simulink library "Arithmetic_Operations_Lib"  (Simulink 8.7)
settings: Solver=ode45  StartTime=0.0  StopTime=10.0  RelTol=1e-3
libraries: Arithmetic_Operations_Lib x56, commutil2 x8
settings Model: Creator=uzivatel  LastModifiedBy=Jozko Mrkvicka

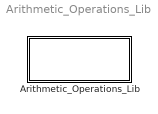
== system Arithmetic_Operations_Lib ==
  Arithmetic_Operations_Lib : Subsystem

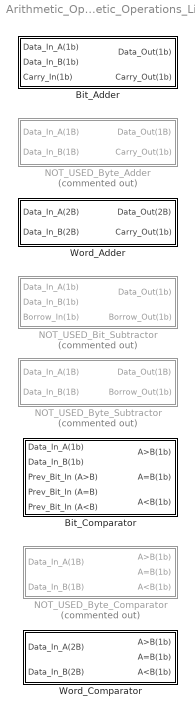
== system Arithmetic_Operations_Lib/Arithmetic_Operations_Lib ==
  Bit_Adder : Subsystem
  Bit_Comparator : Subsystem
  NOT_USED_Bit_Subtractor : Subsystem  Commented=on
  NOT_USED_Byte_Adder : Subsystem  Commented=on
  NOT_USED_Byte_Comparator : Subsystem  Commented=on
  NOT_USED_Byte_Subtractor : Subsystem  Commented=on
  Word_Adder : Subsystem
  Word_Comparator : Subsystem

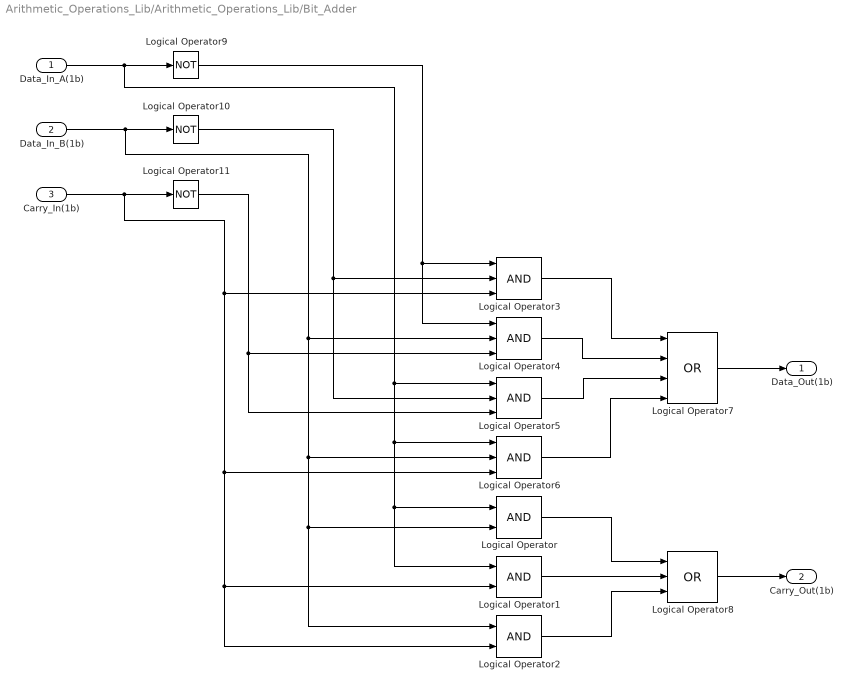
== system Arithmetic_Operations_Lib/Arithmetic_Operations_Lib/Bit_Adder ==
  Data_In_A(1b) : Inport
  Data_In_B(1b) : Inport  Port=2
  Carry_In(1b) : Inport  Port=3
  Logical Operator : Logic  IconShape=distinctive  AllPortsSameDT=off  OutDataTypeStr=boolean
  Logical Operator1 : Logic  IconShape=distinctive  AllPortsSameDT=off  OutDataTypeStr=boolean
  Logical Operator10 : Logic  Operator=NOT  Inputs=4  IconShape=distinctive  AllPortsSameDT=off  OutDataTypeStr=boolean
  Logical Operator11 : Logic  Operator=NOT  Inputs=4  IconShape=distinctive  AllPortsSameDT=off  OutDataTypeStr=boolean
  Logical Operator2 : Logic  IconShape=distinctive  AllPortsSameDT=off  OutDataTypeStr=boolean
  Logical Operator{3..6} (4 alike) : Logic  Inputs=3  IconShape=distinctive  AllPortsSameDT=off  OutDataTypeStr=boolean
  Logical Operator7 : Logic  Operator=OR  Inputs=4  IconShape=distinctive  AllPortsSameDT=off  OutDataTypeStr=boolean
  Logical Operator8 : Logic  Operator=OR  Inputs=3  IconShape=distinctive  AllPortsSameDT=off  OutDataTypeStr=boolean
  Logical Operator9 : Logic  Operator=NOT  Inputs=4  IconShape=distinctive  AllPortsSameDT=off  OutDataTypeStr=boolean
  Data_Out(1b) : Outport
  Carry_Out(1b) : Outport  Port=2
  wires:
  Logical Operator11/1 -> Logical Operator4/3, Logical Operator5/3
  Logical Operator10/1 -> Logical Operator3/2, Logical Operator5/2
  Logical Operator9/1 -> Logical Operator3/1, Logical Operator4/1
  Data_In_A(1b)/1 -> Logical Operator9/1, Logical Operator5/1, Logical Operator6/1, Logical Operator/1, Logical Operator1/1
  Data_In_B(1b)/1 -> Logical Operator10/1, Logical Operator4/2, Logical Operator6/2, Logical Operator/2, Logical Operator2/1
  Carry_In(1b)/1 -> Logical Operator11/1, Logical Operator3/3, Logical Operator6/3, Logical Operator1/2, Logical Operator2/2
  Logical Operator2/1 -> Logical Operator8/3
  Logical Operator1/1 -> Logical Operator8/2
  Logical Operator/1 -> Logical Operator8/1
  Logical Operator8/1 -> Carry_Out(1b)/1
  Logical Operator7/1 -> Data_Out(1b)/1
  Logical Operator6/1 -> Logical Operator7/4
  Logical Operator5/1 -> Logical Operator7/3
  Logical Operator4/1 -> Logical Operator7/2
  Logical Operator3/1 -> Logical Operator7/1

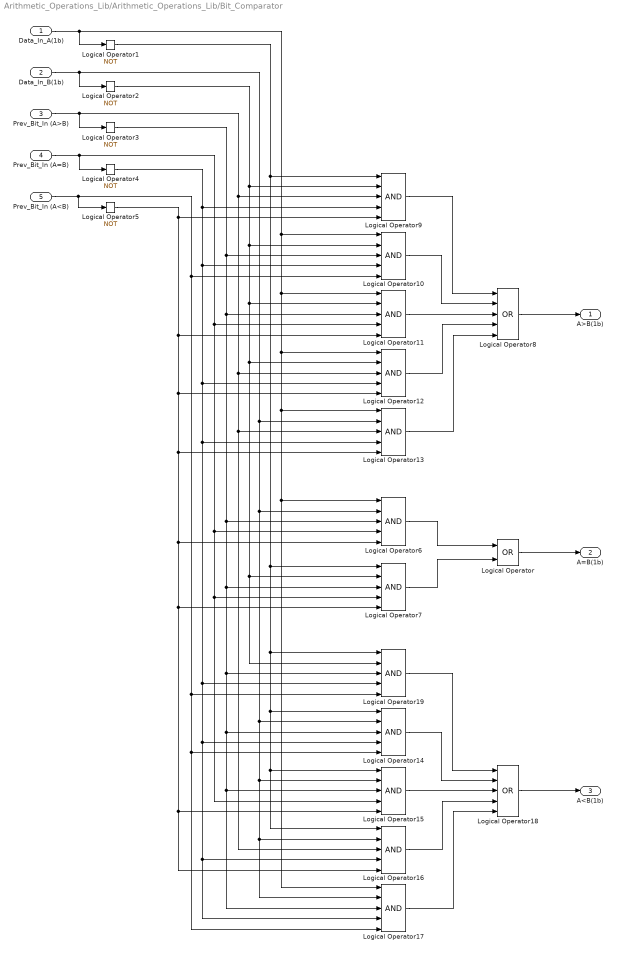
== system Arithmetic_Operations_Lib/Arithmetic_Operations_Lib/Bit_Comparator ==
  Data_In_A(1b) : Inport
  Data_In_B(1b) : Inport  Port=2
  Prev_Bit_In (A>B) : Inport  Port=3
  Prev_Bit_In (A=B) : Inport  Port=4
  Prev_Bit_In (A<B) : Inport  Port=5
  Logical Operator : Logic  Operator=OR  IconShape=distinctive  AllPortsSameDT=off  OutDataTypeStr=boolean
  Logical Operator{1..5} (5 alike) : Logic  Operator=NOT  IconShape=distinctive  AllPortsSameDT=off  OutDataTypeStr=boolean
  Logical Operator{6..7,9..17,19} (12 alike) : Logic  Inputs=5  IconShape=distinctive  AllPortsSameDT=off  OutDataTypeStr=boolean
  Logical Operator18 : Logic  Operator=OR  Inputs=5  IconShape=distinctive  AllPortsSameDT=off  OutDataTypeStr=boolean
  Logical Operator8 : Logic  Operator=OR  Inputs=5  IconShape=distinctive  AllPortsSameDT=off  OutDataTypeStr=boolean
  A>B(1b) : Outport
  A=B(1b) : Outport  Port=2
  A<B(1b) : Outport  Port=3
  wires:
  Logical Operator16/1 -> Logical Operator18/4
  Logical Operator17/1 -> Logical Operator18/5
  Logical Operator19/1 -> Logical Operator18/1
  Logical Operator15/1 -> Logical Operator18/3
  Logical Operator14/1 -> Logical Operator18/2
  Logical Operator4/1 -> Logical Operator9/4, Logical Operator10/4, Logical Operator12/4, Logical Operator13/4, Logical Operator19/4, Logical Operator14/4, Logical Operator17/4, Logical Operator16/4
  Data_In_A(1b)/1 -> Logical Operator10/1, Logical Operator11/1, Logical Operator12/1, Logical Operator13/1, Logical Operator6/1, Logical Operator17/1, Logical Operator1/1
  Logical Operator5/1 -> Logical Operator9/5, Logical Operator11/5, Logical Operator12/5, Logical Operator13/5, Logical Operator6/5, Logical Operator7/5, Logical Operator15/5, Logical Operator16/5
  Logical Operator18/1 -> A<B(1b)/1
  Logical Operator2/1 -> Logical Operator9/2, Logical Operator10/2, Logical Operator11/2, Logical Operator12/2, Logical Operator7/2, Logical Operator19/2
  Logical Operator1/1 -> Logical Operator9/1, Logical Operator7/1, Logical Operator19/1, Logical Operator14/1, Logical Operator15/1, Logical Operator16/1
  Logical Operator3/1 -> Logical Operator10/3, Logical Operator11/3, Logical Operator6/3, Logical Operator7/3, Logical Operator19/3, Logical Operator14/3, Logical Operator15/3, Logical Operator17/3
  Prev_Bit_In (A<B)/1 -> Logical Operator5/1, Logical Operator10/5, Logical Operator19/5, Logical Operator14/5, Logical Operator17/5
  Prev_Bit_In (A>B)/1 -> Logical Operator3/1, Logical Operator9/3, Logical Operator12/3, Logical Operator13/3, Logical Operator16/3
  Prev_Bit_In (A=B)/1 -> Logical Operator11/4, Logical Operator6/4, Logical Operator7/4, Logical Operator15/4, Logical Operator4/1
  Logical Operator6/1 -> Logical Operator/1
  Logical Operator7/1 -> Logical Operator/2
  Data_In_B(1b)/1 -> Logical Operator2/1, Logical Operator13/2, Logical Operator6/2, Logical Operator17/2, Logical Operator16/2, Logical Operator15/2, Logical Operator14/2
  Logical Operator/1 -> A=B(1b)/1
  Logical Operator8/1 -> A>B(1b)/1
  Logical Operator13/1 -> Logical Operator8/5
  Logical Operator11/1 -> Logical Operator8/3
  Logical Operator10/1 -> Logical Operator8/2
  Logical Operator12/1 -> Logical Operator8/4
  Logical Operator9/1 -> Logical Operator8/1

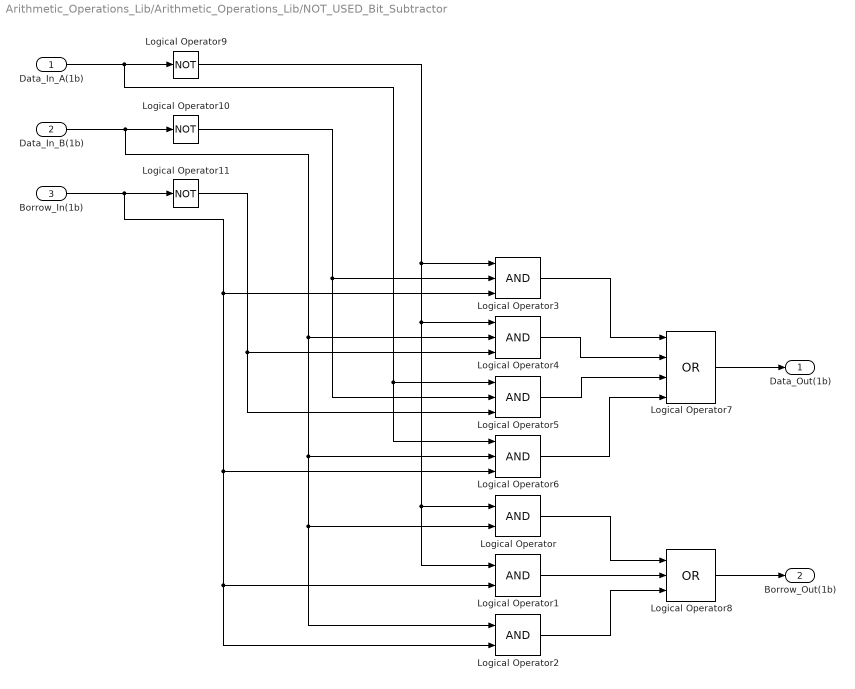
== system Arithmetic_Operations_Lib/Arithmetic_Operations_Lib/NOT_USED_Bit_Subtractor ==
  Data_In_A(1b) : Inport
  Data_In_B(1b) : Inport  Port=2
  Borrow_In(1b) : Inport  Port=3
  Logical Operator : Logic  IconShape=distinctive  AllPortsSameDT=off  OutDataTypeStr=boolean
  Logical Operator1 : Logic  IconShape=distinctive  AllPortsSameDT=off  OutDataTypeStr=boolean
  Logical Operator10 : Logic  Operator=NOT  Inputs=4  IconShape=distinctive  AllPortsSameDT=off  OutDataTypeStr=boolean
  Logical Operator11 : Logic  Operator=NOT  Inputs=4  IconShape=distinctive  AllPortsSameDT=off  OutDataTypeStr=boolean
  Logical Operator2 : Logic  IconShape=distinctive  AllPortsSameDT=off  OutDataTypeStr=boolean
  Logical Operator{3..6} (4 alike) : Logic  Inputs=3  IconShape=distinctive  AllPortsSameDT=off  OutDataTypeStr=boolean
  Logical Operator7 : Logic  Operator=OR  Inputs=4  IconShape=distinctive  AllPortsSameDT=off  OutDataTypeStr=boolean
  Logical Operator8 : Logic  Operator=OR  Inputs=3  IconShape=distinctive  AllPortsSameDT=off  OutDataTypeStr=boolean
  Logical Operator9 : Logic  Operator=NOT  Inputs=4  IconShape=distinctive  AllPortsSameDT=off  OutDataTypeStr=boolean
  Data_Out(1b) : Outport
  Borrow_Out(1b) : Outport  Port=2
  wires:
  Logical Operator11/1 -> Logical Operator4/3, Logical Operator5/3
  Logical Operator10/1 -> Logical Operator3/2, Logical Operator5/2
  Logical Operator9/1 -> Logical Operator3/1, Logical Operator4/1, Logical Operator/1, Logical Operator1/1
  Data_In_A(1b)/1 -> Logical Operator9/1, Logical Operator5/1, Logical Operator6/1
  Data_In_B(1b)/1 -> Logical Operator10/1, Logical Operator4/2, Logical Operator6/2, Logical Operator/2, Logical Operator2/1
  Borrow_In(1b)/1 -> Logical Operator11/1, Logical Operator3/3, Logical Operator6/3, Logical Operator1/2, Logical Operator2/2
  Logical Operator2/1 -> Logical Operator8/3
  Logical Operator1/1 -> Logical Operator8/2
  Logical Operator/1 -> Logical Operator8/1
  Logical Operator8/1 -> Borrow_Out(1b)/1
  Logical Operator7/1 -> Data_Out(1b)/1
  Logical Operator6/1 -> Logical Operator7/4
  Logical Operator5/1 -> Logical Operator7/3
  Logical Operator4/1 -> Logical Operator7/2
  Logical Operator3/1 -> Logical Operator7/1

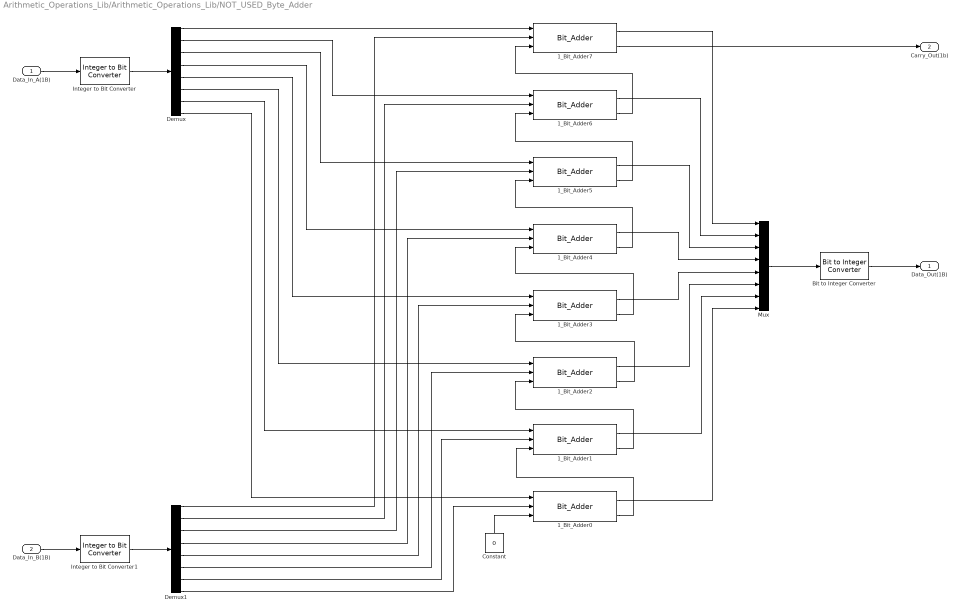
== system Arithmetic_Operations_Lib/Arithmetic_Operations_Lib/NOT_USED_Byte_Adder ==
  Data_In_A(1B) : Inport
  Data_In_B(1B) : Inport  Port=2
  1_Bit_Adder{0..7} (8 alike) : Arithmetic_Operations_Lib/Arithmetic_Operations_Lib/Bit_Adder
  Bit to Integer Converter : commutil2/Bit to Integer Converter  nbits=8  bitOrder=MSB first  signedOutputValues=Unsigned  outDtype=uint8  outDtypeSigned=Inherit via internal rule
  Constant : Constant  Value=0
  Demux : Demux  Outputs=8
  Demux1 : Demux  Outputs=8
  Integer to Bit Converter : commutil2/Integer to Bit Converter  nbits=8  signedInputValues=Unsigned  bitOrder=MSB first  outDtype=uint8
  Integer to Bit Converter1 : commutil2/Integer to Bit Converter  nbits=8  signedInputValues=Unsigned  bitOrder=MSB first  outDtype=uint8
  Mux : Mux  Inputs=8
  Data_Out(1B) : Outport
  Carry_Out(1b) : Outport  Port=2
  wires:
  Bit to Integer Converter/1 -> Data_Out(1B)/1
  Mux/1 -> Bit to Integer Converter/1
  Integer to Bit Converter1/1 -> Demux1/1
  Data_In_B(1B)/1 -> Integer to Bit Converter1/1
  Integer to Bit Converter/1 -> Demux/1
  Data_In_A(1B)/1 -> Integer to Bit Converter/1
  1_Bit_Adder6/2 -> 1_Bit_Adder7/3
  1_Bit_Adder5/2 -> 1_Bit_Adder6/3
  1_Bit_Adder4/2 -> 1_Bit_Adder5/3
  1_Bit_Adder3/2 -> 1_Bit_Adder4/3
  1_Bit_Adder2/2 -> 1_Bit_Adder3/3
  1_Bit_Adder1/2 -> 1_Bit_Adder2/3
  1_Bit_Adder0/2 -> 1_Bit_Adder1/3
  1_Bit_Adder7/2 -> Carry_Out(1b)/1
  Constant/1 -> 1_Bit_Adder0/3
  Demux1/8 -> 1_Bit_Adder0/2
  Demux1/7 -> 1_Bit_Adder1/2
  Demux1/6 -> 1_Bit_Adder2/2
  Demux1/5 -> 1_Bit_Adder3/2
  Demux1/4 -> 1_Bit_Adder4/2
  Demux1/3 -> 1_Bit_Adder5/2
  Demux1/2 -> 1_Bit_Adder6/2
  Demux1/1 -> 1_Bit_Adder7/2
  Demux/8 -> 1_Bit_Adder0/1
  Demux/7 -> 1_Bit_Adder1/1
  Demux/6 -> 1_Bit_Adder2/1
  Demux/5 -> 1_Bit_Adder3/1
  Demux/4 -> 1_Bit_Adder4/1
  Demux/3 -> 1_Bit_Adder5/1
  Demux/2 -> 1_Bit_Adder6/1
  Demux/1 -> 1_Bit_Adder7/1
  1_Bit_Adder3/1 -> Mux/5
  1_Bit_Adder4/1 -> Mux/4
  1_Bit_Adder5/1 -> Mux/3
  1_Bit_Adder2/1 -> Mux/6
  1_Bit_Adder1/1 -> Mux/7
  1_Bit_Adder0/1 -> Mux/8
  1_Bit_Adder6/1 -> Mux/2
  1_Bit_Adder7/1 -> Mux/1

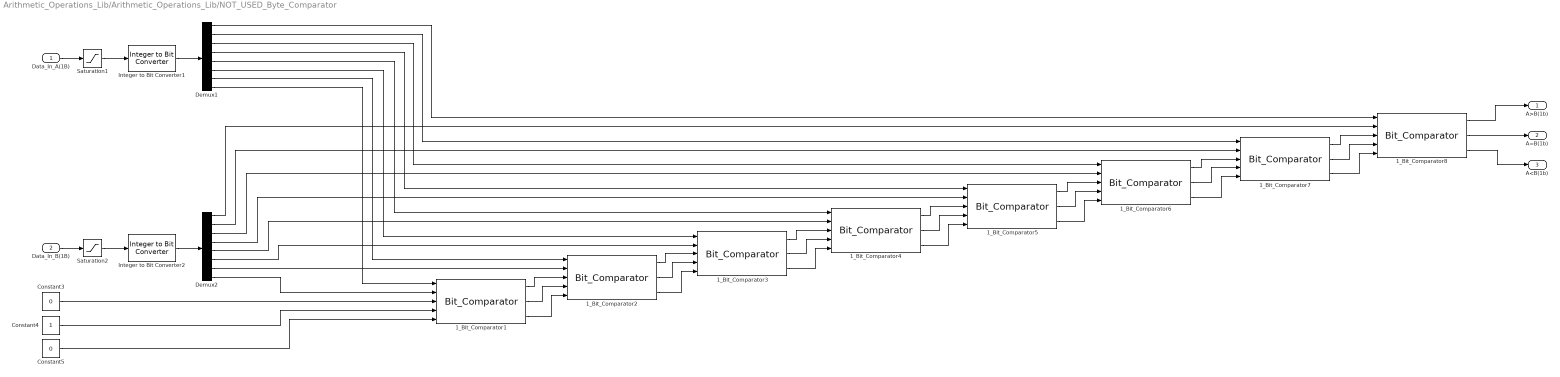
== system Arithmetic_Operations_Lib/Arithmetic_Operations_Lib/NOT_USED_Byte_Comparator ==
  Data_In_A(1B) : Inport
  Data_In_B(1B) : Inport  Port=2
  1_Bit_Comparator{1..8} (8 alike) : Arithmetic_Operations_Lib/Arithmetic_Operations_Lib/Bit_Comparator
  Constant3 : Constant  Value=0  OutDataTypeStr=int16
  Constant4 : Constant  OutDataTypeStr=int16
  Constant5 : Constant  Value=0  OutDataTypeStr=int16
  Demux1 : Demux  Outputs=8
  Demux2 : Demux  Outputs=8
  Integer to Bit Converter1 : commutil2/Integer to Bit Converter  nbits=8  signedInputValues=Unsigned  bitOrder=MSB first  outDtype=uint8
  Integer to Bit Converter2 : commutil2/Integer to Bit Converter  nbits=8  signedInputValues=Unsigned  bitOrder=MSB first  outDtype=uint8
  Saturation1 : Saturate  UpperLimit=255  LowerLimit=0
  Saturation2 : Saturate  UpperLimit=255  LowerLimit=0
  A>B(1b) : Outport
  A=B(1b) : Outport  Port=2
  A<B(1b) : Outport  Port=3
  wires:
  1_Bit_Comparator8/3 -> A<B(1b)/1
  1_Bit_Comparator8/1 -> A>B(1b)/1
  1_Bit_Comparator8/2 -> A=B(1b)/1
  Demux1/1 -> 1_Bit_Comparator8/1
  Demux1/2 -> 1_Bit_Comparator7/1
  Demux1/3 -> 1_Bit_Comparator6/1
  Demux1/4 -> 1_Bit_Comparator5/1
  Demux1/5 -> 1_Bit_Comparator4/1
  Demux1/6 -> 1_Bit_Comparator3/1
  Demux1/7 -> 1_Bit_Comparator2/1
  Data_In_A(1B)/1 -> Saturation1/1
  Saturation1/1 -> Integer to Bit Converter1/1
  Integer to Bit Converter1/1 -> Demux1/1
  Demux2/1 -> 1_Bit_Comparator8/2
  Demux2/2 -> 1_Bit_Comparator7/2
  Demux2/3 -> 1_Bit_Comparator6/2
  Demux2/4 -> 1_Bit_Comparator5/2
  Demux2/5 -> 1_Bit_Comparator4/2
  Demux2/6 -> 1_Bit_Comparator3/2
  Demux2/7 -> 1_Bit_Comparator2/2
  Data_In_B(1B)/1 -> Saturation2/1
  Saturation2/1 -> Integer to Bit Converter2/1
  Integer to Bit Converter2/1 -> Demux2/1
  1_Bit_Comparator7/3 -> 1_Bit_Comparator8/5
  1_Bit_Comparator7/2 -> 1_Bit_Comparator8/4
  1_Bit_Comparator7/1 -> 1_Bit_Comparator8/3
  1_Bit_Comparator6/3 -> 1_Bit_Comparator7/5
  1_Bit_Comparator6/2 -> 1_Bit_Comparator7/4
  1_Bit_Comparator6/1 -> 1_Bit_Comparator7/3
  1_Bit_Comparator5/3 -> 1_Bit_Comparator6/5
  1_Bit_Comparator5/2 -> 1_Bit_Comparator6/4
  1_Bit_Comparator5/1 -> 1_Bit_Comparator6/3
  1_Bit_Comparator4/3 -> 1_Bit_Comparator5/5
  1_Bit_Comparator4/2 -> 1_Bit_Comparator5/4
  1_Bit_Comparator4/1 -> 1_Bit_Comparator5/3
  1_Bit_Comparator3/3 -> 1_Bit_Comparator4/5
  1_Bit_Comparator3/2 -> 1_Bit_Comparator4/4
  1_Bit_Comparator3/1 -> 1_Bit_Comparator4/3
  1_Bit_Comparator2/3 -> 1_Bit_Comparator3/5
  1_Bit_Comparator2/1 -> 1_Bit_Comparator3/3
  1_Bit_Comparator2/2 -> 1_Bit_Comparator3/4
  Demux1/8 -> 1_Bit_Comparator1/1
  1_Bit_Comparator1/3 -> 1_Bit_Comparator2/5
  Demux2/8 -> 1_Bit_Comparator1/2
  Constant3/1 -> 1_Bit_Comparator1/3
  1_Bit_Comparator1/1 -> 1_Bit_Comparator2/3
  1_Bit_Comparator1/2 -> 1_Bit_Comparator2/4
  Constant5/1 -> 1_Bit_Comparator1/5
  Constant4/1 -> 1_Bit_Comparator1/4

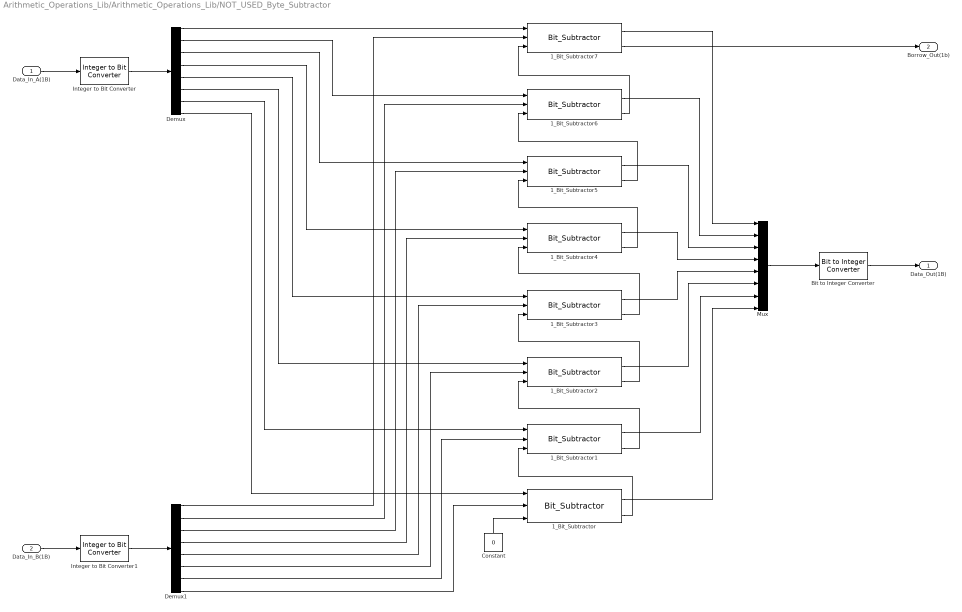
== system Arithmetic_Operations_Lib/Arithmetic_Operations_Lib/NOT_USED_Byte_Subtractor ==
  Data_In_A(1B) : Inport
  Data_In_B(1B) : Inport  Port=2
  1_Bit_Subtractor{,1..7} (8 alike) : Arithmetic_Operations_Lib/Arithmetic_Operations_Lib/Bit_Subtractor
  Bit to Integer Converter : commutil2/Bit to Integer Converter  nbits=8  bitOrder=MSB first  signedOutputValues=Unsigned  outDtype=uint8  outDtypeSigned=Inherit via internal rule
  Constant : Constant  Value=0
  Demux : Demux  Outputs=8
  Demux1 : Demux  Outputs=8
  Integer to Bit Converter : commutil2/Integer to Bit Converter  nbits=8  signedInputValues=Unsigned  bitOrder=MSB first  outDtype=uint8
  Integer to Bit Converter1 : commutil2/Integer to Bit Converter  nbits=8  signedInputValues=Unsigned  bitOrder=MSB first  outDtype=uint8
  Mux : Mux  Inputs=8
  Data_Out(1B) : Outport
  Borrow_Out(1b) : Outport  Port=2
  wires:
  Bit to Integer Converter/1 -> Data_Out(1B)/1
  Mux/1 -> Bit to Integer Converter/1
  Integer to Bit Converter1/1 -> Demux1/1
  Data_In_B(1B)/1 -> Integer to Bit Converter1/1
  Integer to Bit Converter/1 -> Demux/1
  Data_In_A(1B)/1 -> Integer to Bit Converter/1
  1_Bit_Subtractor6/2 -> 1_Bit_Subtractor7/3
  1_Bit_Subtractor5/2 -> 1_Bit_Subtractor6/3
  1_Bit_Subtractor4/2 -> 1_Bit_Subtractor5/3
  1_Bit_Subtractor3/2 -> 1_Bit_Subtractor4/3
  1_Bit_Subtractor2/2 -> 1_Bit_Subtractor3/3
  1_Bit_Subtractor1/2 -> 1_Bit_Subtractor2/3
  1_Bit_Subtractor/2 -> 1_Bit_Subtractor1/3
  1_Bit_Subtractor7/2 -> Borrow_Out(1b)/1
  Constant/1 -> 1_Bit_Subtractor/3
  Demux1/8 -> 1_Bit_Subtractor/2
  Demux1/7 -> 1_Bit_Subtractor1/2
  Demux1/6 -> 1_Bit_Subtractor2/2
  Demux1/5 -> 1_Bit_Subtractor3/2
  Demux1/4 -> 1_Bit_Subtractor4/2
  Demux1/3 -> 1_Bit_Subtractor5/2
  Demux1/2 -> 1_Bit_Subtractor6/2
  Demux1/1 -> 1_Bit_Subtractor7/2
  Demux/8 -> 1_Bit_Subtractor/1
  Demux/7 -> 1_Bit_Subtractor1/1
  Demux/6 -> 1_Bit_Subtractor2/1
  Demux/5 -> 1_Bit_Subtractor3/1
  Demux/4 -> 1_Bit_Subtractor4/1
  Demux/3 -> 1_Bit_Subtractor5/1
  Demux/2 -> 1_Bit_Subtractor6/1
  Demux/1 -> 1_Bit_Subtractor7/1
  1_Bit_Subtractor3/1 -> Mux/5
  1_Bit_Subtractor4/1 -> Mux/4
  1_Bit_Subtractor5/1 -> Mux/3
  1_Bit_Subtractor2/1 -> Mux/6
  1_Bit_Subtractor1/1 -> Mux/7
  1_Bit_Subtractor/1 -> Mux/8
  1_Bit_Subtractor6/1 -> Mux/2
  1_Bit_Subtractor7/1 -> Mux/1

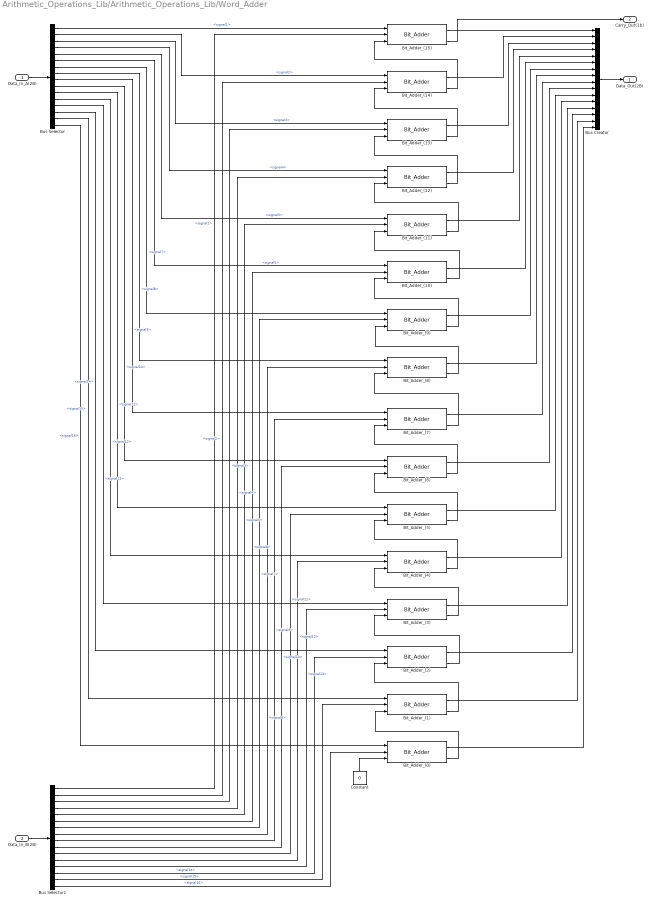
== system Arithmetic_Operations_Lib/Arithmetic_Operations_Lib/Word_Adder ==
  Data_In_A(2B) : Inport
  Data_In_B(2B) : Inport  Port=2
  Bit_Adder_(0) : Arithmetic_Operations_Lib/Arithmetic_Operations_Lib/Bit_Adder
  Bit_Adder_(1) : Arithmetic_Operations_Lib/Arithmetic_Operations_Lib/Bit_Adder
  Bit_Adder_(10) : Arithmetic_Operations_Lib/Arithmetic_Operations_Lib/Bit_Adder
  Bit_Adder_(11) : Arithmetic_Operations_Lib/Arithmetic_Operations_Lib/Bit_Adder
  Bit_Adder_(12) : Arithmetic_Operations_Lib/Arithmetic_Operations_Lib/Bit_Adder
  Bit_Adder_(13) : Arithmetic_Operations_Lib/Arithmetic_Operations_Lib/Bit_Adder
  Bit_Adder_(14) : Arithmetic_Operations_Lib/Arithmetic_Operations_Lib/Bit_Adder
  Bit_Adder_(15) : Arithmetic_Operations_Lib/Arithmetic_Operations_Lib/Bit_Adder
  Bit_Adder_(2) : Arithmetic_Operations_Lib/Arithmetic_Operations_Lib/Bit_Adder
  Bit_Adder_(3) : Arithmetic_Operations_Lib/Arithmetic_Operations_Lib/Bit_Adder
  Bit_Adder_(4) : Arithmetic_Operations_Lib/Arithmetic_Operations_Lib/Bit_Adder
  Bit_Adder_(5) : Arithmetic_Operations_Lib/Arithmetic_Operations_Lib/Bit_Adder
  Bit_Adder_(6) : Arithmetic_Operations_Lib/Arithmetic_Operations_Lib/Bit_Adder
  Bit_Adder_(7) : Arithmetic_Operations_Lib/Arithmetic_Operations_Lib/Bit_Adder
  Bit_Adder_(8) : Arithmetic_Operations_Lib/Arithmetic_Operations_Lib/Bit_Adder
  Bit_Adder_(9) : Arithmetic_Operations_Lib/Arithmetic_Operations_Lib/Bit_Adder
  Bus Creator : BusCreator  Inputs=16
  Bus Selector : BusSelector  OutputSignals=signal1,signal2,signal3,signal4,signal5,signal6,signal7,signal8,signal9,signal10,signal11,signal12,signal13,signal14,signal15,signal16
  Bus Selector1 : BusSelector  OutputSignals=signal1,signal2,signal3,signal4,signal5,signal6,signal7,signal8,signal9,signal10,signal11,signal12,signal13,signal14,signal15,signal16
  Constant : Constant  Value=0
  Data_Out(2B) : Outport
  Carry_Out(1b) : Outport  Port=2
  wires:
  Bit_Adder_(6)/2 -> Bit_Adder_(7)/3
  Bit_Adder_(5)/2 -> Bit_Adder_(6)/3
  Bit_Adder_(4)/2 -> Bit_Adder_(5)/3
  Bit_Adder_(3)/2 -> Bit_Adder_(4)/3
  Bit_Adder_(2)/2 -> Bit_Adder_(3)/3
  Bit_Adder_(1)/2 -> Bit_Adder_(2)/3
  Bit_Adder_(0)/2 -> Bit_Adder_(1)/3
  Bit_Adder_(7)/2 -> Bit_Adder_(8)/3
  Constant/1 -> Bit_Adder_(0)/3
  Bus Selector1/16 -> Bit_Adder_(0)/2  "<signal16>"
  Bus Selector1/15 -> Bit_Adder_(1)/2  "<signal15>"
  Bus Selector1/14 -> Bit_Adder_(2)/2  "<signal14>"
  Bus Selector1/13 -> Bit_Adder_(3)/2  "<signal13>"
  Bus Selector1/12 -> Bit_Adder_(4)/2  "<signal12>"
  Bus Selector1/11 -> Bit_Adder_(5)/2  "<signal11>"
  Bus Selector1/10 -> Bit_Adder_(6)/2  "<signal10>"
  Bus Selector1/9 -> Bit_Adder_(7)/2  "<signal9>"
  Bus Selector/16 -> Bit_Adder_(0)/1  "<signal16>"
  Bus Selector/15 -> Bit_Adder_(1)/1  "<signal15>"
  Bus Selector/14 -> Bit_Adder_(2)/1  "<signal14>"
  Bus Selector/13 -> Bit_Adder_(3)/1  "<signal13>"
  Bus Selector/12 -> Bit_Adder_(4)/1  "<signal12>"
  Bus Selector/11 -> Bit_Adder_(5)/1  "<signal11>"
  Bus Selector/10 -> Bit_Adder_(6)/1  "<signal10>"
  Bus Selector/9 -> Bit_Adder_(7)/1  "<signal9>"
  Bit_Adder_(3)/1 -> Bus Creator/13
  Bit_Adder_(4)/1 -> Bus Creator/12
  Bit_Adder_(5)/1 -> Bus Creator/11
  Bit_Adder_(2)/1 -> Bus Creator/14
  Bit_Adder_(1)/1 -> Bus Creator/15
  Bit_Adder_(0)/1 -> Bus Creator/16
  Bit_Adder_(6)/1 -> Bus Creator/10
  Bit_Adder_(7)/1 -> Bus Creator/9
  Bus Creator/1 -> Data_Out(2B)/1
  Data_In_B(2B)/1 -> Bus Selector1/1
  Data_In_A(2B)/1 -> Bus Selector/1
  Bit_Adder_(14)/2 -> Bit_Adder_(15)/3
  Bit_Adder_(13)/2 -> Bit_Adder_(14)/3
  Bit_Adder_(12)/2 -> Bit_Adder_(13)/3
  Bit_Adder_(11)/2 -> Bit_Adder_(12)/3
  Bit_Adder_(10)/2 -> Bit_Adder_(11)/3
  Bit_Adder_(9)/2 -> Bit_Adder_(10)/3
  Bit_Adder_(8)/2 -> Bit_Adder_(9)/3
  Bit_Adder_(15)/2 -> Carry_Out(1b)/1
  Bit_Adder_(15)/1 -> Bus Creator/1
  Bit_Adder_(14)/1 -> Bus Creator/2
  Bit_Adder_(13)/1 -> Bus Creator/3
  Bit_Adder_(12)/1 -> Bus Creator/4
  Bit_Adder_(11)/1 -> Bus Creator/5
  Bit_Adder_(10)/1 -> Bus Creator/6
  Bit_Adder_(9)/1 -> Bus Creator/7
  Bit_Adder_(8)/1 -> Bus Creator/8
  Bus Selector1/8 -> Bit_Adder_(8)/2  "<signal8>"
  Bus Selector1/7 -> Bit_Adder_(9)/2  "<signal7>"
  Bus Selector1/6 -> Bit_Adder_(10)/2  "<signal6>"
  Bus Selector1/5 -> Bit_Adder_(11)/2  "<signal5>"
  Bus Selector1/4 -> Bit_Adder_(12)/2  "<signal4>"
  Bus Selector1/3 -> Bit_Adder_(13)/2  "<signal3>"
  Bus Selector1/2 -> Bit_Adder_(14)/2  "<signal2>"
  Bus Selector1/1 -> Bit_Adder_(15)/2  "<signal1>"
  Bus Selector/1 -> Bit_Adder_(15)/1  "<signal1>"
  Bus Selector/2 -> Bit_Adder_(14)/1  "<signal2>"
  Bus Selector/3 -> Bit_Adder_(13)/1  "<signal3>"
  Bus Selector/4 -> Bit_Adder_(12)/1  "<signal4>"
  Bus Selector/5 -> Bit_Adder_(11)/1  "<signal5>"
  Bus Selector/6 -> Bit_Adder_(10)/1  "<signal6>"
  Bus Selector/7 -> Bit_Adder_(9)/1  "<signal7>"
  Bus Selector/8 -> Bit_Adder_(8)/1  "<signal8>"

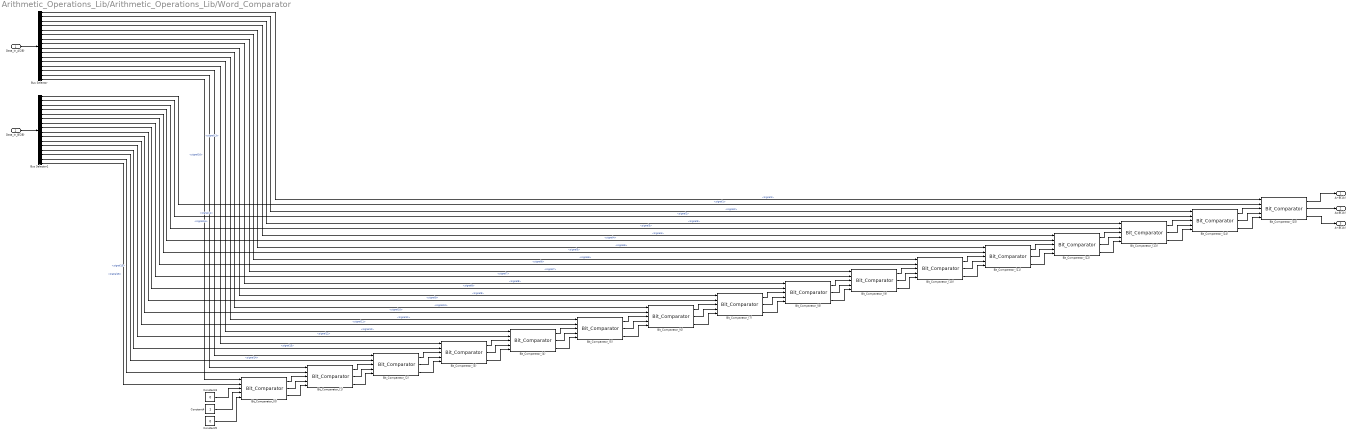
== system Arithmetic_Operations_Lib/Arithmetic_Operations_Lib/Word_Comparator ==
  Data_In_A(2B) : Inport
  Data_In_B(2B) : Inport  Port=2
  Bit_Comparator_(0) : Arithmetic_Operations_Lib/Arithmetic_Operations_Lib/Bit_Comparator
  Bit_Comparator_(1) : Arithmetic_Operations_Lib/Arithmetic_Operations_Lib/Bit_Comparator
  Bit_Comparator_(10) : Arithmetic_Operations_Lib/Arithmetic_Operations_Lib/Bit_Comparator
  Bit_Comparator_(11) : Arithmetic_Operations_Lib/Arithmetic_Operations_Lib/Bit_Comparator
  Bit_Comparator_(12) : Arithmetic_Operations_Lib/Arithmetic_Operations_Lib/Bit_Comparator
  Bit_Comparator_(13) : Arithmetic_Operations_Lib/Arithmetic_Operations_Lib/Bit_Comparator
  Bit_Comparator_(14) : Arithmetic_Operations_Lib/Arithmetic_Operations_Lib/Bit_Comparator
  Bit_Comparator_(15) : Arithmetic_Operations_Lib/Arithmetic_Operations_Lib/Bit_Comparator
  Bit_Comparator_(2) : Arithmetic_Operations_Lib/Arithmetic_Operations_Lib/Bit_Comparator
  Bit_Comparator_(3) : Arithmetic_Operations_Lib/Arithmetic_Operations_Lib/Bit_Comparator
  Bit_Comparator_(4) : Arithmetic_Operations_Lib/Arithmetic_Operations_Lib/Bit_Comparator
  Bit_Comparator_(5) : Arithmetic_Operations_Lib/Arithmetic_Operations_Lib/Bit_Comparator
  Bit_Comparator_(6) : Arithmetic_Operations_Lib/Arithmetic_Operations_Lib/Bit_Comparator
  Bit_Comparator_(7) : Arithmetic_Operations_Lib/Arithmetic_Operations_Lib/Bit_Comparator
  Bit_Comparator_(8) : Arithmetic_Operations_Lib/Arithmetic_Operations_Lib/Bit_Comparator
  Bit_Comparator_(9) : Arithmetic_Operations_Lib/Arithmetic_Operations_Lib/Bit_Comparator
  Bus Selector : BusSelector  OutputSignals=signal1,signal2,signal3,signal4,signal5,signal6,signal7,signal8,signal9,signal10,signal11,signal12,signal13,signal14,signal15,signal16
  Bus Selector1 : BusSelector  OutputSignals=signal1,signal2,signal3,signal4,signal5,signal6,signal7,signal8,signal9,signal10,signal11,signal12,signal13,signal14,signal15,signal16
  Constant3 : Constant  Value=0  OutDataTypeStr=int16
  Constant4 : Constant  OutDataTypeStr=int16
  Constant5 : Constant  Value=0  OutDataTypeStr=int16
  A>B(1b) : Outport
  A=B(1b) : Outport  Port=2
  A<B(1b) : Outport  Port=3
  wires:
  Bit_Comparator_(7)/3 -> Bit_Comparator_(8)/5
  Bit_Comparator_(7)/1 -> Bit_Comparator_(8)/3
  Bit_Comparator_(7)/2 -> Bit_Comparator_(8)/4
  Bus Selector/9 -> Bit_Comparator_(7)/1  "<signal9>"
  Bus Selector/10 -> Bit_Comparator_(6)/1  "<signal10>"
  Bus Selector/11 -> Bit_Comparator_(5)/1  "<signal11>"
  Bus Selector/12 -> Bit_Comparator_(4)/1  "<signal12>"
  Bus Selector/13 -> Bit_Comparator_(3)/1  "<signal13>"
  Bus Selector/14 -> Bit_Comparator_(2)/1  "<signal14>"
  Bus Selector/15 -> Bit_Comparator_(1)/1  "<signal15>"
  Data_In_A(2B)/1 -> Bus Selector/1
  Bus Selector1/9 -> Bit_Comparator_(7)/2  "<signal9>"
  Bus Selector1/10 -> Bit_Comparator_(6)/2  "<signal10>"
  Bus Selector1/11 -> Bit_Comparator_(5)/2  "<signal11>"
  Bus Selector1/12 -> Bit_Comparator_(4)/2  "<signal12>"
  Bus Selector1/13 -> Bit_Comparator_(3)/2  "<signal13>"
  Bus Selector1/14 -> Bit_Comparator_(2)/2  "<signal14>"
  Bus Selector1/15 -> Bit_Comparator_(1)/2  "<signal15>"
  Data_In_B(2B)/1 -> Bus Selector1/1
  Bit_Comparator_(6)/3 -> Bit_Comparator_(7)/5
  Bit_Comparator_(6)/2 -> Bit_Comparator_(7)/4
  Bit_Comparator_(6)/1 -> Bit_Comparator_(7)/3
  Bit_Comparator_(5)/3 -> Bit_Comparator_(6)/5
  Bit_Comparator_(5)/2 -> Bit_Comparator_(6)/4
  Bit_Comparator_(5)/1 -> Bit_Comparator_(6)/3
  Bit_Comparator_(4)/3 -> Bit_Comparator_(5)/5
  Bit_Comparator_(4)/2 -> Bit_Comparator_(5)/4
  Bit_Comparator_(4)/1 -> Bit_Comparator_(5)/3
  Bit_Comparator_(3)/3 -> Bit_Comparator_(4)/5
  Bit_Comparator_(3)/2 -> Bit_Comparator_(4)/4
  Bit_Comparator_(3)/1 -> Bit_Comparator_(4)/3
  Bit_Comparator_(2)/3 -> Bit_Comparator_(3)/5
  Bit_Comparator_(2)/2 -> Bit_Comparator_(3)/4
  Bit_Comparator_(2)/1 -> Bit_Comparator_(3)/3
  Bit_Comparator_(1)/3 -> Bit_Comparator_(2)/5
  Bit_Comparator_(1)/1 -> Bit_Comparator_(2)/3
  Bit_Comparator_(1)/2 -> Bit_Comparator_(2)/4
  Bus Selector/16 -> Bit_Comparator_(0)/1  "<signal16>"
  Bit_Comparator_(0)/3 -> Bit_Comparator_(1)/5
  Bus Selector1/16 -> Bit_Comparator_(0)/2  "<signal16>"
  Constant3/1 -> Bit_Comparator_(0)/3
  Bit_Comparator_(0)/1 -> Bit_Comparator_(1)/3
  Bit_Comparator_(0)/2 -> Bit_Comparator_(1)/4
  Constant5/1 -> Bit_Comparator_(0)/5
  Constant4/1 -> Bit_Comparator_(0)/4
  Bit_Comparator_(15)/3 -> A<B(1b)/1
  Bit_Comparator_(15)/1 -> A>B(1b)/1
  Bit_Comparator_(15)/2 -> A=B(1b)/1
  Bus Selector/1 -> Bit_Comparator_(15)/1  "<signal1>"
  Bus Selector/2 -> Bit_Comparator_(14)/1  "<signal2>"
  Bus Selector/3 -> Bit_Comparator_(13)/1  "<signal3>"
  Bus Selector/4 -> Bit_Comparator_(12)/1  "<signal4>"
  Bus Selector/5 -> Bit_Comparator_(11)/1  "<signal5>"
  Bus Selector/6 -> Bit_Comparator_(10)/1  "<signal6>"
  Bus Selector/7 -> Bit_Comparator_(9)/1  "<signal7>"
  Bus Selector1/1 -> Bit_Comparator_(15)/2  "<signal1>"
  Bus Selector1/2 -> Bit_Comparator_(14)/2  "<signal2>"
  Bus Selector1/3 -> Bit_Comparator_(13)/2  "<signal3>"
  Bus Selector1/4 -> Bit_Comparator_(12)/2  "<signal4>"
  Bus Selector1/5 -> Bit_Comparator_(11)/2  "<signal5>"
  Bus Selector1/6 -> Bit_Comparator_(10)/2  "<signal6>"
  Bus Selector1/7 -> Bit_Comparator_(9)/2  "<signal7>"
  Bit_Comparator_(14)/3 -> Bit_Comparator_(15)/5
  Bit_Comparator_(14)/2 -> Bit_Comparator_(15)/4
  Bit_Comparator_(14)/1 -> Bit_Comparator_(15)/3
  Bit_Comparator_(13)/3 -> Bit_Comparator_(14)/5
  Bit_Comparator_(13)/2 -> Bit_Comparator_(14)/4
  Bit_Comparator_(13)/1 -> Bit_Comparator_(14)/3
  Bit_Comparator_(12)/3 -> Bit_Comparator_(13)/5
  Bit_Comparator_(12)/2 -> Bit_Comparator_(13)/4
  Bit_Comparator_(12)/1 -> Bit_Comparator_(13)/3
  Bit_Comparator_(11)/3 -> Bit_Comparator_(12)/5
  Bit_Comparator_(11)/2 -> Bit_Comparator_(12)/4
  Bit_Comparator_(11)/1 -> Bit_Comparator_(12)/3
  Bit_Comparator_(10)/3 -> Bit_Comparator_(11)/5
  Bit_Comparator_(10)/2 -> Bit_Comparator_(11)/4
  Bit_Comparator_(10)/1 -> Bit_Comparator_(11)/3
  Bit_Comparator_(9)/3 -> Bit_Comparator_(10)/5
  Bit_Comparator_(9)/1 -> Bit_Comparator_(10)/3
  Bit_Comparator_(9)/2 -> Bit_Comparator_(10)/4
  Bit_Comparator_(8)/3 -> Bit_Comparator_(9)/5
  Bit_Comparator_(8)/1 -> Bit_Comparator_(9)/3
  Bit_Comparator_(8)/2 -> Bit_Comparator_(9)/4
  Bus Selector/8 -> Bit_Comparator_(8)/1  "<signal8>"
  Bus Selector1/8 -> Bit_Comparator_(8)/2  "<signal8>"
